simulink model "task12"  (R2022b)
settings: Solver=FixedStepAuto  StartTime=0.0  StopTime=7  RelTol=1e-8
undefined symbols (not defined in the file): k0, k1, lambda1, lambda2, T, y0, y1
libraries: simulink_extras x3
settings Model: Creator=anton  LastModifiedBy=anton
settings DataIOCC: ExternalInput=data

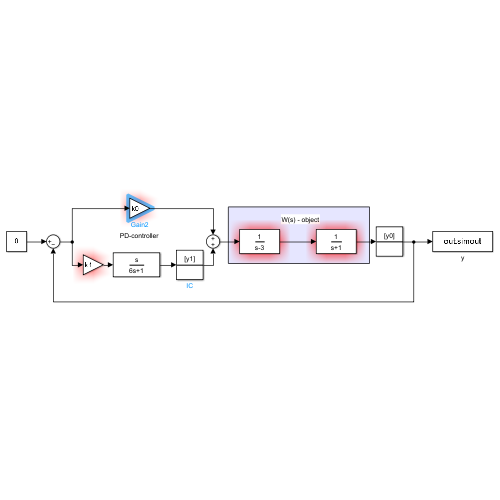
[thumbnail: Simulink's stored preview of the top-level diagram]
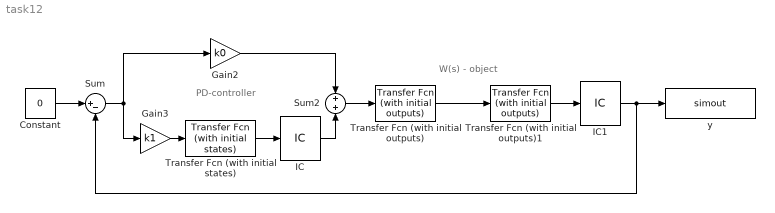
== system task12 ==
  note: W(s) - object
  note: PD-controller
  Constant : Constant  Value=0
  Gain2 : Gain  Gain=k0
  Gain3 : Gain  Gain=k1
  IC : InitialCondition  Value=y1
  IC1 : InitialCondition  Value=y0
  Sum : Sum  Inputs=|+-
  Sum2 : Sum
  Transfer Fcn (with initial outputs) : simulink_extras/Additional Linear/Transfer Fcn (with initial outputs)  N=[1]  D=[1 -lambda1]  Y0=0  U0=0
  Transfer Fcn (with initial outputs)1 : simulink_extras/Additional Linear/Transfer Fcn (with initial outputs)  N=[1]  D=[1 -lambda2]  Y0=0  U0=0
  Transfer Fcn (with initial states) : simulink_extras/Additional Linear/Transfer Fcn (with initial states)  N=[1 0]  D=[T 1]  X0=[y0 y1]
  y : ToWorkspace  VariableName=simout  SaveFormat=Timeseries  SampleTime=-1
  wires:
  Constant/1 -> Sum/1
  Transfer Fcn (with initial outputs)1/1 -> IC1/1
  Transfer Fcn (with initial states)/1 -> IC/1
  Gain3/1 -> Transfer Fcn (with initial states)/1
  Gain2/1 -> Sum2/1
  Sum2/1 -> Transfer Fcn (with initial outputs)/1
  Transfer Fcn (with initial outputs)/1 -> Transfer Fcn (with initial outputs)1/1
  Sum/1 -> Gain2/1, Gain3/1
  IC1/1 -> Sum/2, y/1
  IC/1 -> Sum2/2
